simulink model "ElectricalSystem_Test"  (R2019b)
settings: Solver=VariableStepAuto  StartTime=0.0  StopTime=inf  RelTol=1e-3
PostLoadFcn:
  | set_up_test_model
undefined symbols (not defined in the file): AC1CB, AC2CB, AirSupplyIC, APSCB, ATCCabActivation, ATCZeroSpeed, ATOTBDemand, Audio, BLCB, Braking, CECB, CELCB, Class, CMCCB, CRSBCB, CSACB, CSBCB, CSCCB, DeadmanSafetyDevice, DIOCB1, DIOCB2, DLCB, DMICB, Doors, DPLCB, DRCB, EIVIB, ElectricalSystemInput, ElectricalTrainConnection, ElectricalUnitConnection, EmergencyBrakePB, Enabled, ForwardDirection, GrossMass, HasCab, HasMainCompressor, HasMotor, HasPanto, HeadlightSwitch, Height, HLCB, HornPB, ILCB1, ILCB2, IsDM1, IsDM2, IsM1, IsM2, IsT1, IsT2, LeftSideDoorOpen, Length, LoadingMass, MainReservoirPressureSwitch, MasterKeySwitch, MaxVehicles, ModeSelector, NotImmobilise, NotSafetyBrake, NVICB ... (+47)
libraries: TestBenchLib x81
(part 1 of 2)
settings Model: EnablePacing=on  Creator=jwang  LastModifiedBy=ext-nadpurob
settings DebuggingCC: FrameProcessingCompatibilityMsg=warning  ArithmeticOperatorsInVariantConditions=warning
settings SFSimCC: SimUseLocalCustomCode=off  CustomCodeUndefinedFunction=UseInterfaceOnly
settings RTWCC: RTWUseLocalCustomCode=off
settings CodeAppCC: StateflowObjectComments=on

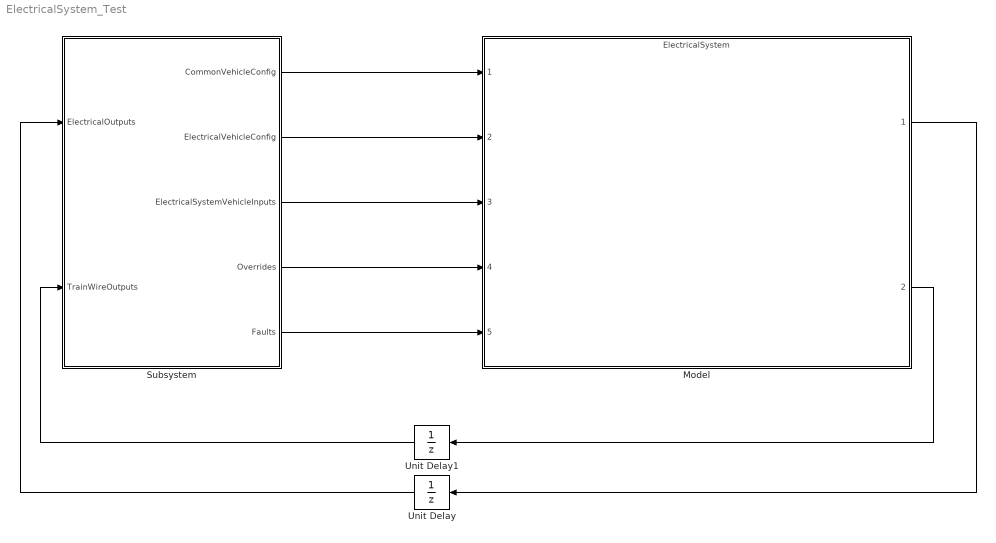
== system ElectricalSystem_Test ==
  Model : ModelReference  ModelNameDialog=ElectricalSystem.slx  ParameterArgumentNames=Prm_ElectricalSystem  ParameterArgumentValues=[Z_ElectricalSystemPrm]  UsingDefaultArgumentValue=0  SimulationMode=Normal  ModelReferenceVersion=1.1522
  Subsystem : Subsystem
  Unit Delay : UnitDelay  SampleTime=-1  HasFrameUpgradeWarning=on
  Unit Delay1 : UnitDelay  SampleTime=-1  HasFrameUpgradeWarning=on
  wires:
  Subsystem/1(CommonVehicleConfig) -> Model/1
  Subsystem/2(ElectricalVehicleConfig) -> Model/2
  Subsystem/3(ElectricalSystemVehicleInputs) -> Model/3
  Subsystem/4(Overrides) -> Model/4
  Subsystem/5(Faults) -> Model/5
  Model/2 -> Unit Delay1/1
  Model/1 -> Unit Delay/1
  Unit Delay/1 -> Subsystem/1(ElectricalOutputs)
  Unit Delay1/1 -> Subsystem/2(TrainWireOutputs)

== system ElectricalSystem_Test/Subsystem ==
  ElectricalOutputs : Inport
  TrainWireOutputs : Inport  Port=2
  Common Config Creator For Testing : Subsystem
  Data Store Memory : DataStoreMemory  DataStoreName=ElectricalSystemInput  ReadBeforeWriteMsg=warning  WriteAfterWriteMsg=warning  WriteAfterReadMsg=warning  InitialValue=zeros(1, MaxVehicles)  ShowAdditionalParam=off  OutDataTypeStr=Bus: BD_ElectricalSystem_In_Vehicle  Dimensions=MaxVehicles
  Data Store Memory1 : DataStoreMemory  DataStoreName=Faults  ReadBeforeWriteMsg=warning  WriteAfterWriteMsg=warning  WriteAfterReadMsg=warning  InitialValue=zeros(1, MaxVehicles)  ShowAdditionalParam=off  OutDataTypeStr=Bus: BD_ElectricalSystem_In_Faults  Dimensions=MaxVehicles
  Data Store Read : DataStoreRead  DataStoreName=ElectricalSystemInput
  Data Store Read1 : DataStoreRead  DataStoreName=Faults
  Data Store Write9 : DataStoreWrite  DataStoreName=ElectricalSystemInput  DataStoreElements=ElectricalSystemInput(1).ModelStatus.IsInitialized#ElectricalSystemInput(2).ModelStatus.IsInitialized#ElectricalSystemInput(3).ModelStatus.IsInitialized#ElectricalSystemInput(4).ModelStatus.IsInitialized#ElectricalSystemInput(5).ModelStatus.IsInitialized#ElectricalSystemInput(6).ModelStatus.IsInitialized
  Data Type Conversion78 : DataTypeConversion
  Electrical Config Creator For Testing : Subsystem
  Overrides1 : Subsystem
  Step : Step  SampleTime=0
  Testing : Subsystem
  CommonVehicleConfig : Outport
  ElectricalVehicleConfig : Outport  Port=2
  ElectricalSystemVehicleInputs : Outport  Port=3
  Overrides : Outport  Port=4
  Faults : Outport  Port=5
  wires:
  Common Config Creator For Testing/1(CommonVehicleConfig) -> CommonVehicleConfig/1
  Electrical Config Creator For Testing/1(ElectricalVehicleConfig) -> ElectricalVehicleConfig/1
  Overrides1/1(Override) -> Overrides/1
  Data Store Read1/1 -> Faults/1
  Data Store Read/1 -> ElectricalSystemVehicleInputs/1
  ElectricalOutputs/1 -> Testing/1(ElectricalSystemVehicleOut)
  TrainWireOutputs/1 -> Testing/2(TrainWireOutput)
  Step/1 -> Data Type Conversion78/1
  Data Type Conversion78/1 -> Data Store Write9/6, Data Store Write9/5, Data Store Write9/4, Data Store Write9/3, Data Store Write9/2, Data Store Write9/1

== system ElectricalSystem_Test/Subsystem/Common Config Creator For Testing ==
  Orientation : Constant  Value=[1 1 1 2 2 2]
  Subsystem : Subsystem
  CommonVehicleConfig : Outport  VectorParamsAs1DForOutWhenUnconnected=off
  wires:
  Orientation/1 -> Subsystem/1(Orientation)
  Subsystem/1(Out1) -> CommonVehicleConfig/1

== system ElectricalSystem_Test/Subsystem/Electrical Config Creator For Testing ==
  HasAirCompressor : Constant  Value=[1,0,0,0,0,1]  OutDataTypeStr=boolean
  HasCab : Constant  Value=[1,0,0,0,0,1]  OutDataTypeStr=boolean
  HasMotor : Constant  Value=[1,0,1,1,0,1]  OutDataTypeStr=boolean
  HasPanto : Constant  Value=[0,1,0,0,1,0]  OutDataTypeStr=boolean
  IsDM1 : Constant  Value=[1,0,0,0,0,0]  OutDataTypeStr=boolean
  IsDM2 : Constant  Value=[0,0,0,0,0,1]  OutDataTypeStr=boolean
  IsM1 : Constant  Value=[0,0,1,0,0,0]  OutDataTypeStr=boolean
  IsM2 : Constant  Value=[0,0,0,1,0,0]  OutDataTypeStr=boolean
  IsT1 : Constant  Value=[0,1,0,0,0,0]  OutDataTypeStr=boolean
  IsT2 : Constant  Value=[0,0,0,0,1,0]  OutDataTypeStr=boolean
  Subsystem : Subsystem
  ElectricalVehicleConfig : Outport  VectorParamsAs1DForOutWhenUnconnected=off
  wires:
  Subsystem/1(Out1) -> ElectricalVehicleConfig/1
  IsDM1/1 -> Subsystem/1(IsDM1)
  IsT2/1 -> Subsystem/5(isT2)
  IsDM2/1 -> Subsystem/6(IsDM2)
  HasPanto/1 -> Subsystem/7(HasPanto)
  HasCab/1 -> Subsystem/8(HasCab)
  HasMotor/1 -> Subsystem/9(HasMotor)
  HasAirCompressor/1 -> Subsystem/10(HasMainCompressor)
  IsM2/1 -> Subsystem/4(IsM2)
  IsM1/1 -> Subsystem/3(IsM1)
  IsT1/1 -> Subsystem/2(IsT1)

== system ElectricalSystem_Test/Subsystem/Overrides1 ==
  Constant : Constant  Value=zeros(1,MaxVehicles)  OutDataTypeStr=Bus: BD_ElectricalSystem_In_Overrides
  Override : Outport  VectorParamsAs1DForOutWhenUnconnected=off
  wires:
  Constant/1 -> Override/1

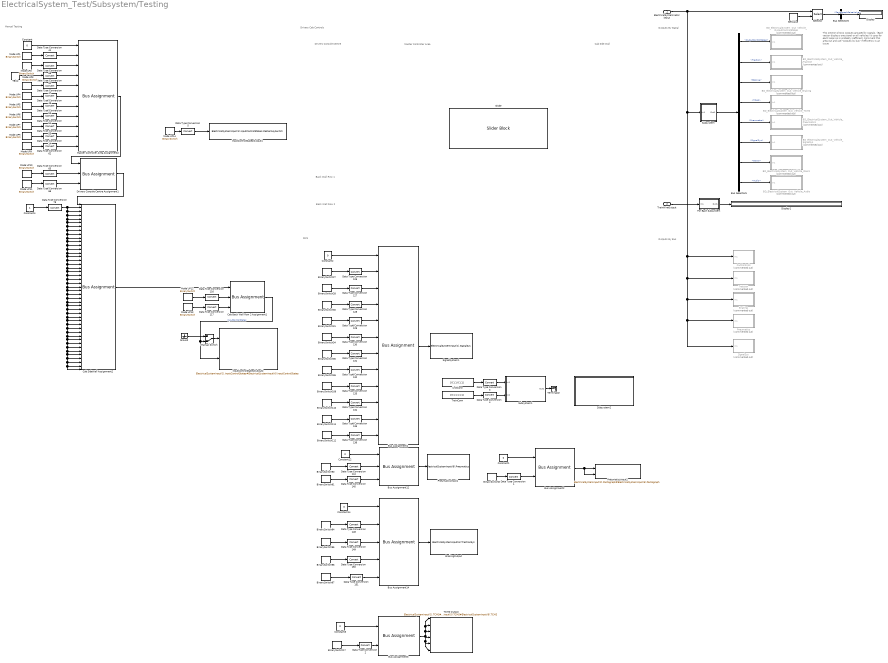
== system ElectricalSystem_Test/Subsystem/Testing ==
  note: This section shows outputs grouped by signals.
      | (Each vector displays one signal on all vehicles)
      | It uses for each loops so is probably inefficient.
      |
      | Comment this area out and use "outputs by bus" if
      | efficiency is an issue
  note: Manual Testing
  note: Outputs By Signal
  note: Drivers Cab Controls
  note: Back Wall Row 2
  note: Back Wall Row 1
  note: Cab Side Wall
  note: Drivers Console Centre
  note: Master Controller Area
  note: DM1
  note: Outputs By Bus
  ElectricalSystemVehicleOut : Inport
  TrainWireOutput : Inport  Port=2
  BD_ElectricalSystem_Out_Vehicle_Audio : Subsystem  Commented=on
  BD_ElectricalSystem_Out_Vehicle_Braking : Subsystem  Commented=on
  BD_ElectricalSystem_Out_Vehicle_Doors : Subsystem  Commented=on
  BD_ElectricalSystem_Out_Vehicle_OutputControlStates : Subsystem  Commented=on
  BD_ElectricalSystem_Out_Vehicle_Pneumatics : Subsystem  Commented=on
  BD_ElectricalSystem_Out_Vehicle_SignalSys : Subsystem  Commented=on
  BD_ElectricalSystem_Out_Vehicle_TCMS : Subsystem  Commented=on
  BD_ElectricalSystem_Out_Vehicle_Traction : Subsystem  Commented=on
  BinarySwitch{8,17,27..28,30..31,34..36,90..91,94..97,109..112} (19 alike) : TestBenchLib/BinarySwitch  value=0  init_value=0  block_colour=[0 1 0]  WorkspaceVarName=0
      settings: SourceProductName=Sydac Utilities
  Braking : Subsystem  Commented=on
  BrakingOutput : DataStoreWrite  DataStoreName=ElectricalSystemInput  DataStoreElements=ElectricalSystemInput(6).TractionSys
  Bus Assignment1 : BusAssignment  AssignedSignals=NotImmobilise,ATCZeroSpeed,NotSafetyBrake,LeftSideDoorOpen,RightSideDoorOpen,WakeUpCommand,UTOPBIndicator,UTOModeActive,ATCCabActivation,ATOTBDemand,TractionForward
  Bus Assignment12 : BusAssignment  AssignedSignals=MainReservoirPressureSwitch,PantographPressureSwitch
  Bus Assignment14 : BusAssignment  AssignedSignals=ForwardDirection,ReverseDirection,TCU_KStatus,TCU_AKStatus
  Bus Assignment2 : BusAssignment  AssignedSignals=PantographPosition
  Bus Assignment3 : BusAssignment  AssignedSignals=Overspeed
  Bus Selector5 : BusSelector  OutputSignals=OutputControlStates,Traction,Braking,TCMS,Pneumatics,SignalSys,Doors,Audio
  Bus Selector6 : BusSelector  OutputSignals=Pneumatics.PantographRaiseValve
  Cab Back Wall Row 2 Assignment1 : BusAssignment  AssignedSignals=ParkBrakeApplyPB,ParkBrakeReleasePB
  Cab SideWall Assignment2 : BusAssignment  AssignedSignals=CMCCB,RIO1CB,RIO2CB,TDICB,DIOCB2,DIOCB1,CSCCB,CSBCB,CSACB,CECB,UCCB,BLCB,CRSBCB,DMICB,NVICB,VIO1CB,VIO2CB,APSCB,DLCB,DRCB,DPLCB,HLCB,TLCB,CELCB,ILCB1,ILCB2,PANCB,TBCCB1,TBCCB2,POCB,TVDUCB,ODDCB,WFLCB,WWCB,VCBCCB,PADCB,SAC1CCB,SAC2CCB,AC1CB,AC2CB,RCCB,SFB,EIVIB,AirSupplyIC
  Constant : Constant  Value=0  OutDataTypeStr=Bus: BD_ElectricalSystem_In_Vehicle_InputControlStates
  Constant1 : Constant  Value=0  OutDataTypeStr=Bus: BD_ElectricalSystem_In_Vehicle_Pantograph
  Constant12 : Constant  Value=0  OutDataTypeStr=Bus: BD_ElectricalSystem_In_Vehicle_Pneumatics
  Constant14 : Constant  Value=0  OutDataTypeStr=Bus: BD_ElectricalSystem_In_Vehicle_Traction
  Constant2 : Constant  Value=0  OutDataTypeStr=Bus: BD_ElectricalSystem_In_Vehicle_SignalSys
  Constant3 : Constant  Value=0  OutDataTypeStr=Bus: BD_ElectricalSystem_In_Vehicle_TCMS
  Constant4 : Constant
  Data Type Conversion{1..5,14,41..42,47,49,53..55,58,62,65..66,78,116..117,126..136,144..145,148..151} (37 alike) : DataTypeConversion
  Display : Display
  Display1 : Display
  Drivers Console Centre Assignment1 : BusAssignment  AssignedSignals=EmergencyBrakePB,HornPB
  For Each Subsystem : Subsystem  TreatAsAtomicUnit=on
  Ground : Ground
  InputControlStatesOutput1 : DataStoreWrite  DataStoreName=ElectricalSystemInput  DataStoreElements=ElectricalSystemInput(1).InputControlStates.MasterKeySwitch
  InputControlStatesOutput2 : DataStoreWrite  DataStoreName=ElectricalSystemInput  DataStoreElements=ElectricalSystemInput(1).InputControlStates#ElectricalSystemInput(6).InputControlStates
  Manual Switch : ManualSwitch  CurrentSetting=0
  Master Controller Area Assignment2 : BusAssignment  AssignedSignals=MasterKeySwitch,PowerONPB,TractionBrakeController,VCBOpenPB,VCBClosePB,ParkBrakeReleasePB,DeadmanSafetyDevice,ModeSelector,WiperSwitch,HeadlightSwitch
  Mode UP{1..14} (14 alike) : TestBenchLib/BinarySwitch  value=0  init_value=0  block_colour=[0 1 0]  WorkspaceVarName=0
      settings: SourceProductName=Sydac Utilities
  OutControls : Subsystem  Commented=on
  Pneumatics : Subsystem  Commented=on
  PneumaticsInput1 : DataStoreWrite  DataStoreName=ElectricalSystemInput  DataStoreElements=ElectricalSystemInput(6).Pneumatics
  PneumaticsInput2 : DataStoreWrite  DataStoreName=ElectricalSystemInput  DataStoreElements=ElectricalSystemInput(2).Pantograph#ElectricalSystemInput(5).Pantograph
  Selector : Selector  InputPortWidth=6  IndexOptions=Index vector (port)  Indices=[1 3]  OutputSizes=1
  SetValue : TestBenchLib/SetValue  value=1  init_value=1  WorkspaceVarName=0
      settings: SourceProductName=Sydac Utilities
  SignalSys : Subsystem  Commented=on
  SignalSystem1 : DataStoreWrite  DataStoreName=ElectricalSystemInput  DataStoreElements=ElectricalSystemInput(1).SignalSys
  Slider : SliderBlock  ScaleMin=-101
  Subsystem : Subsystem
  Subsystem1 : Subsystem
  Subsystem2 : Subsystem
  TBC2 : TestBenchLib/SetValue  value=19.57995345744682  init_value=19.57995345744682  WorkspaceVarName=0
      settings: SourceProductName=Sydac Utilities
  TCMS Output : DataStoreWrite  DataStoreName=ElectricalSystemInput  DataStoreElements=ElectricalSystemInput(1).TCMS#ElectricalSystemInput(2).TCMS#ElectricalSystemInput(3).TCMS#ElectricalSystemInput(4).TCMS#ElectricalSystemInput(5).TCMS#ElectricalSystemInput(6).TCMS
  Terminator : Terminator
  Traction : Subsystem  Commented=on
  TrainConn : Constant  Value=[0 1 1 1 1 1]
  UnitConn : Constant  Value=[0 1 1 0 1 1]
  wires:
  Bus Selector5/1 -> BD_ElectricalSystem_Out_Vehicle_OutputControlStates/1(In1)  "<OutputControlStates>"
  Bus Selector5/2 -> BD_ElectricalSystem_Out_Vehicle_Traction/1(In1)  "<Traction>"
  Bus Selector5/3 -> BD_ElectricalSystem_Out_Vehicle_Braking/1(In1)  "<Braking>"
  Bus Selector5/4 -> BD_ElectricalSystem_Out_Vehicle_TCMS/1(In1)  "<TCMS>"
  Bus Selector5/5 -> BD_ElectricalSystem_Out_Vehicle_Pneumatics/1(In1)  "<Pneumatics>"
  Bus Selector5/6 -> BD_ElectricalSystem_Out_Vehicle_SignalSys/1(In1)  "<SignalSys>"
  Bus Selector5/7 -> BD_ElectricalSystem_Out_Vehicle_Doors/1(In1)  "<Doors>"
  ElectricalSystemVehicleOut/1 -> SignalSys/1(In1), Pneumatics/1(In1), Braking/1(In1), Traction/1(In1), OutControls/1(In1), Subsystem/1(In1), Selector/1
  Subsystem/1(Out1) -> Bus Selector5/1
  Master Controller Area Assignment2/1 -> Drivers Console Centre Assignment1/1
  Mode UP6/1 -> Data Type Conversion54/1
  Mode UP3/1 -> Data Type Conversion47/1
  Mode UP7/1 -> Data Type Conversion55/1
  Mode UP5/1 -> Data Type Conversion53/1
  Mode UP8/1 -> Data Type Conversion14/1
  Mode UP4/1 -> Data Type Conversion49/1
  TBC2/1 -> Data Type Conversion42/1
  Mode UP9/1 -> Data Type Conversion62/1
  Constant/1 -> Master Controller Area Assignment2/1
  Data Type Conversion41/1 -> Master Controller Area Assignment2/2
  Data Type Conversion58/1 -> Master Controller Area Assignment2/3
  Data Type Conversion42/1 -> Master Controller Area Assignment2/4
  Data Type Conversion47/1 -> Master Controller Area Assignment2/5
  Data Type Conversion49/1 -> Master Controller Area Assignment2/6
  Data Type Conversion53/1 -> Master Controller Area Assignment2/7
  Data Type Conversion54/1 -> Master Controller Area Assignment2/8
  Data Type Conversion55/1 -> Master Controller Area Assignment2/9
  Data Type Conversion14/1 -> Master Controller Area Assignment2/10
  Data Type Conversion62/1 -> Master Controller Area Assignment2/11
  Mode UP11/1 -> Data Type Conversion66/1
  Mode UP10/1 -> Data Type Conversion65/1
  Data Type Conversion65/1 -> Drivers Console Centre Assignment1/2
  Data Type Conversion66/1 -> Drivers Console Centre Assignment1/3
  Constant4/1 -> Data Type Conversion78/1
  Drivers Console Centre Assignment1/1 -> Cab SideWall Assignment2/1
  Data Type Conversion78/1 -> Cab SideWall Assignment2/3, Cab SideWall Assignment2/4, Cab SideWall Assignment2/5, Cab SideWall Assignment2/6, Cab SideWall Assignment2/7, Cab SideWall Assignment2/8, Cab SideWall Assignment2/9, Cab SideWall Assignment2/10, Cab SideWall Assignment2/11, Cab SideWall Assignment2/12, Cab SideWall Assignment2/13, Cab SideWall Assignment2/14, Cab SideWall Assignment2/15, Cab SideWall Assignment2/16, Cab SideWall Assignment2/17, Cab SideWall Assignment2/18, Cab SideWall Assignment2/19, Cab SideWall Assignment2/20, Cab SideWall Assignment2/21, Cab SideWall Assignment2/22, Cab SideWall Assignment2/23, Cab SideWall Assignment2/24, Cab SideWall Assignment2/25, Cab SideWall Assignment2/26, Cab SideWall Assignment2/27, Cab SideWall Assignment2/28, Cab SideWall Assignment2/29, Cab SideWall Assignment2/30, Cab SideWall Assignment2/31, Cab SideWall Assignment2/32, Cab SideWall Assignment2/33, Cab SideWall Assignment2/34, Cab SideWall Assignment2/35, Cab SideWall Assignment2/36, Cab SideWall Assignment2/37, Cab SideWall Assignment2/38, Cab SideWall Assignment2/39, Cab SideWall Assignment2/40, Cab SideWall Assignment2/41, Cab SideWall Assignment2/42, Cab SideWall Assignment2/43, Cab SideWall Assignment2/44, Cab SideWall Assignment2/45, Cab SideWall Assignment2/2
  Cab SideWall Assignment2/1 -> Cab Back Wall Row 2 Assignment1/1
  Mode UP13/1 -> Data Type Conversion117/1
  Mode UP12/1 -> Data Type Conversion116/1
  Cab Back Wall Row 2 Assignment1/1 -> Manual Switch/2, InputControlStatesOutput2/2  "InputControlStates"
  Data Type Conversion116/1 -> Cab Back Wall Row 2 Assignment1/2
  Data Type Conversion117/1 -> Cab Back Wall Row 2 Assignment1/3
  Constant2/1 -> Bus Assignment1/1
  BinarySwitch35/1 -> Data Type Conversion131/1
  BinarySwitch34/1 -> Data Type Conversion130/1
  BinarySwitch31/1 -> Data Type Conversion129/1
  BinarySwitch28/1 -> Data Type Conversion127/1
  BinarySwitch30/1 -> Data Type Conversion128/1
  BinarySwitch27/1 -> Data Type Conversion126/1
  Data Type Conversion126/1 -> Bus Assignment1/2
  Data Type Conversion127/1 -> Bus Assignment1/3
  Data Type Conversion128/1 -> Bus Assignment1/4
  Data Type Conversion129/1 -> Bus Assignment1/5
  Data Type Conversion130/1 -> Bus Assignment1/6
  Data Type Conversion131/1 -> Bus Assignment1/7
  BinarySwitch36/1 -> Data Type Conversion132/1
  BinarySwitch110/1 -> Data Type Conversion134/1
  BinarySwitch109/1 -> Data Type Conversion133/1
  BinarySwitch111/1 -> Data Type Conversion135/1
  BinarySwitch112/1 -> Data Type Conversion136/1
  Data Type Conversion132/1 -> Bus Assignment1/8
  Data Type Conversion133/1 -> Bus Assignment1/9
  Data Type Conversion134/1 -> Bus Assignment1/10
  Data Type Conversion135/1 -> Bus Assignment1/11
  Data Type Conversion136/1 -> Bus Assignment1/12
  Bus Assignment1/1 -> SignalSystem1/1
  Constant12/1 -> Bus Assignment12/1
  BinarySwitch90/1 -> Data Type Conversion144/1
  BinarySwitch91/1 -> Data Type Conversion145/1
  Data Type Conversion144/1 -> Bus Assignment12/2
  Data Type Conversion145/1 -> Bus Assignment12/3
  Bus Assignment12/1 -> PneumaticsInput1/1
  Constant14/1 -> Bus Assignment14/1
  BinarySwitch95/1 -> Data Type Conversion149/1
  BinarySwitch94/1 -> Data Type Conversion148/1
  Data Type Conversion148/1 -> Bus Assignment14/2
  Data Type Conversion149/1 -> Bus Assignment14/3
  BinarySwitch97/1 -> Data Type Conversion151/1
  BinarySwitch96/1 -> Data Type Conversion150/1
  Data Type Conversion150/1 -> Bus Assignment14/4
  Data Type Conversion151/1 -> Bus Assignment14/5
  Bus Assignment14/1 -> BrakingOutput/1
  SetValue/1 -> Selector/2
  Selector/1 -> Bus Selector6/1
  Bus Selector6/1 -> Display/1  "<PantographRaiseValve>"
  Bus Assignment2/1 -> PneumaticsInput2/2, PneumaticsInput2/1
  Constant1/1 -> Bus Assignment2/1
  BinarySwitch8/1 -> Data Type Conversion1/1
  Data Type Conversion1/1 -> Bus Assignment2/2
  Constant3/1 -> Bus Assignment3/1
  Bus Assignment3/1 -> TCMS Output/6, TCMS Output/5, TCMS Output/4, TCMS Output/2, TCMS Output/1, TCMS Output/3
  BinarySwitch17/1 -> Data Type Conversion2/1
  Data Type Conversion2/1 -> Bus Assignment3/2
  Bus Selector5/8 -> BD_ElectricalSystem_Out_Vehicle_Audio/1(In1)  "<Audio>"
  Manual Switch/1 -> InputControlStatesOutput2/1
  Mode UP1/1 -> Data Type Conversion41/1
  Mode UP2/1 -> Data Type Conversion58/1
  TrainWireOutput/1 -> For Each Subsystem/1(In1)
  For Each Subsystem/1(Out1) -> Display1/1
  TrainConn/1 -> Data Type Conversion4/1
  UnitConn/1 -> Data Type Conversion3/1
  Data Type Conversion3/1 -> Subsystem1/1(In1)
  Data Type Conversion4/1 -> Subsystem1/2(In2)
  Subsystem1/1(Out1) -> Terminator/1
  Data Type Conversion5/1 -> InputControlStatesOutput1/1
  Mode UP14/1 -> Data Type Conversion5/1
  Ground/1 -> Manual Switch/1

== system ElectricalSystem_Test/Subsystem/Common Config Creator For Testing/Subsystem ==
  Orientation : Inport  Partition=on  PartitionDimension=1  PartitionWidth=1  PartitionOffset=0
  Bus Assignment : BusAssignment  AssignedSignals=Enabled,Class,Orientation,Length,Height,Width,TareMass,GrossMass,LoadingMass,WheelDiameter
  Constant : Constant  Value=0  OutDataTypeStr=Bus: BD_CommonTrain_Cfg_Vehicle
  Constant1 : Constant
  Data Type Conversion : DataTypeConversion
  For Each : ForEach  DisableCoverage=on
  Ground : Ground
  Out1 : Outport  ConcatenationDimension=1  VectorParamsAs1DForOutWhenUnconnected=off
  wires:
  Constant/1 -> Bus Assignment/1
  Bus Assignment/1 -> Out1/1
  Orientation/1 -> Bus Assignment/4  "Orientation"
  Constant1/1 -> Data Type Conversion/1  "Enabled"
  Data Type Conversion/1 -> Bus Assignment/2
  Ground/1 -> Bus Assignment/11, Bus Assignment/10, Bus Assignment/9, Bus Assignment/8, Bus Assignment/7, Bus Assignment/6, Bus Assignment/5, Bus Assignment/3

== system ElectricalSystem_Test/Subsystem/Electrical Config Creator For Testing/Subsystem ==
  IsDM1 : Inport  Partition=on  PartitionDimension=1  PartitionWidth=1  PartitionOffset=0
  IsT1 : Inport  Port=2  Partition=on  PartitionDimension=1  PartitionWidth=1  PartitionOffset=0
  IsM1 : Inport  Port=3  Partition=on  PartitionDimension=1  PartitionWidth=1  PartitionOffset=0
  IsM2 : Inport  Port=4  Partition=on  PartitionDimension=1  PartitionWidth=1  PartitionOffset=0
  isT2 : Inport  Port=5  Partition=on  PartitionDimension=1  PartitionWidth=1  PartitionOffset=0
  IsDM2 : Inport  Port=6  Partition=on  PartitionDimension=1  PartitionWidth=1  PartitionOffset=0
  HasPanto : Inport  Port=7  Partition=on  PartitionDimension=1  PartitionWidth=1  PartitionOffset=0
  HasCab : Inport  Port=8  Partition=on  PartitionDimension=1  PartitionWidth=1  PartitionOffset=0
  HasMotor : Inport  Port=9  Partition=on  PartitionDimension=1  PartitionWidth=1  PartitionOffset=0
  HasMainCompressor : Inport  Port=10  Partition=on  PartitionDimension=1  PartitionWidth=1  PartitionOffset=0
  Bus Assignment : BusAssignment  AssignedSignals=IsDM1,IsT1,IsM1,IsM2,IsT2,IsDM2,HasPanto,HasCab,HasMotor,HasMainCompressor
  Constant : Constant  Value=0  OutDataTypeStr=Bus: BD_ElectricalSystem_Cfg_Vehicle
  For Each : ForEach  DisableCoverage=on
  Out1 : Outport  ConcatenationDimension=1  VectorParamsAs1DForOutWhenUnconnected=off
  wires:
  IsDM1/1 -> Bus Assignment/2
  Bus Assignment/1 -> Out1/1
  Constant/1 -> Bus Assignment/1
  IsT1/1 -> Bus Assignment/3
  IsM1/1 -> Bus Assignment/4
  IsM2/1 -> Bus Assignment/5
  isT2/1 -> Bus Assignment/6
  IsDM2/1 -> Bus Assignment/7
  HasPanto/1 -> Bus Assignment/8
  HasCab/1 -> Bus Assignment/9
  HasMotor/1 -> Bus Assignment/10
  HasMainCompressor/1 -> Bus Assignment/11

== system ElectricalSystem_Test/Subsystem/Testing/BD_ElectricalSystem_Out_Vehicle_Audio ==
  note: Tc1
  note: M1
  note: Mp1
  note: M3
  note: Mp3
  note: M2
  note: Tc2
  note: Mp2
  note: Tc1
  note: Mp1
  note: M1
  note: Mp3
  note: M3
  note: M2
  note: Mp2
  note: Tc2
  In1 : Inport
  ExtractData : Subsystem  TreatAsAtomicUnit=on
  Pwr{,1..3} (4 alike) : Display
  wires:
  In1/1 -> ExtractData/1(In1)
  ExtractData/1(Out1) -> Pwr/1
  ExtractData/2(Out2) -> Pwr1/1
  ExtractData/3(Out3) -> Pwr2/1
  ExtractData/4(Out4) -> Pwr3/1

== system ElectricalSystem_Test/Subsystem/Testing/BD_ElectricalSystem_Out_Vehicle_Braking ==
  note: ScopyBois
  note: Tc1
  note: Mp1
  note: M1
  note: Mp3
  note: M3
  note: M2
  note: Mp2
  note: Tc2
  note: Tc1
  note: Mp1
  note: M1
  note: Mp3
  note: M3
  note: M2
  note: Mp2
  note: Tc2
  In1 : Inport
  ExtractData : Subsystem  TreatAsAtomicUnit=on
  Pwr{,1..3,6..9} (8 alike) : Display
  wires:
  ExtractData/1(Power) -> Pwr/1
  In1/1 -> ExtractData/1(In1)
  ExtractData/2(Traction) -> Pwr1/1
  ExtractData/3(Braking) -> Pwr2/1
  ExtractData/4(Not High Braking) -> Pwr3/1
  ExtractData/5(Force Brake Release Cmd) -> Pwr6/1
  ExtractData/6(Backup Mode) -> Pwr7/1
  ExtractData/7(NoEB) -> Pwr8/1
  ExtractData/8(NoEB1) -> Pwr9/1

== system ElectricalSystem_Test/Subsystem/Testing/BD_ElectricalSystem_Out_Vehicle_Doors ==
  note: Tc2
  note: Mp2
  note: M2
  note: M3
  note: Mp3
  note: M1
  note: Mp1
  note: Tc1
  note: Mp2
  note: Tc2
  note: M2
  note: Mp3
  note: M3
  note: Mp1
  note: M1
  note: Tc1
  In1 : Inport
  ExtractData : Subsystem  TreatAsAtomicUnit=on
  Pwr{,1..7} (8 alike) : Display
  wires:
  ExtractData/8(Out8) -> Pwr7/1
  ExtractData/7(Out7) -> Pwr6/1
  ExtractData/6(Out6) -> Pwr5/1
  ExtractData/5(Out5) -> Pwr4/1
  ExtractData/4(Out4) -> Pwr3/1
  ExtractData/3(Out3) -> Pwr2/1
  ExtractData/2(Out2) -> Pwr1/1
  ExtractData/1(Out1) -> Pwr/1
  In1/1 -> ExtractData/1(In1)

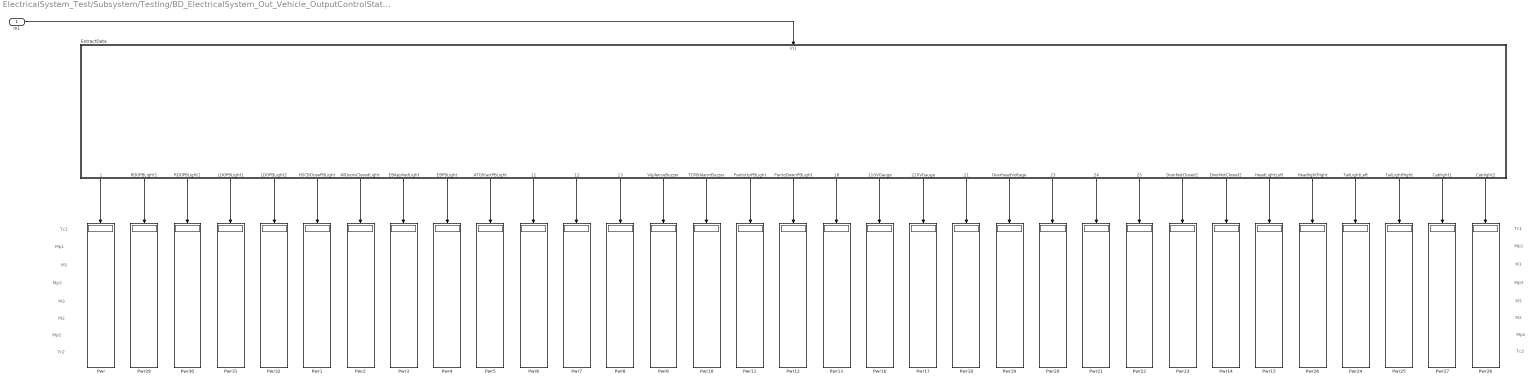
== system ElectricalSystem_Test/Subsystem/Testing/BD_ElectricalSystem_Out_Vehicle_OutputControlStates ==
  note: Tc1
  note: M1
  note: Mp1
  note: M3
  note: Mp3
  note: M2
  note: Tc2
  note: Mp2
  note: Tc1
  note: Mp1
  note: M1
  note: Mp3
  note: M3
  note: M2
  note: Mp2
  note: Tc2
  In1 : Inport
  ExtractData : Subsystem  TreatAsAtomicUnit=on
  Pwr{,1..32} (33 alike) : Display
  wires:
  ExtractData/16(PantoUpPBLight) -> Pwr11/1
  ExtractData/15(TCMSAlarmBuzzer) -> Pwr10/1
  ExtractData/14(VigilanceBuzzer) -> Pwr9/1
  ExtractData/13(DualPressureGaugeBacklight) -> Pwr8/1
  ExtractData/12(BrakeCylinderPressureGauge) -> Pwr7/1
  ExtractData/11(MainReservoirPipePressureGauge) -> Pwr6/1
  ExtractData/10(ATOStartPBLight) -> Pwr5/1
  ExtractData/9(EBPBLight) -> Pwr4/1
  ExtractData/8(EBAppliedLight) -> Pwr3/1
  ExtractData/7(AllDoorsClosedLight) -> Pwr2/1
  ExtractData/6(HSCBClosePBLight) -> Pwr1/1
  ExtractData/1(AutomaticChangeEndPBLight) -> Pwr/1
  In1/1 -> ExtractData/1(In1)
  ExtractData/18(ParkBrakeApplyPBLight) -> Pwr13/1
  ExtractData/19(110VGauge) -> Pwr16/1
  ExtractData/20(220VGauge) -> Pwr17/1
  ExtractData/21(DualBatteryGaugeBacklight) -> Pwr18/1
  ExtractData/22(OverheadVoltage) -> Pwr19/1
  ExtractData/23(OverheadVoltageBacklight) -> Pwr20/1
  ExtractData/24(PneumaticBrakesNotReleased1) -> Pwr21/1
  ExtractData/25(PneumaticBrakesNotReleased2) -> Pwr22/1
  ExtractData/26(DoorNotClosed1) -> Pwr23/1
  ExtractData/27(DoorNotClosed2) -> Pwr14/1
  ExtractData/28(HeadLightLeft) -> Pwr15/1
  ExtractData/29(HeadlightRight) -> Pwr26/1
  ExtractData/30(TailLightLeft) -> Pwr24/1
  ExtractData/17(PantoDownPBLight) -> Pwr12/1
  ExtractData/31(TailLightRight) -> Pwr25/1
  ExtractData/32(Cablight1) -> Pwr27/1
  ExtractData/33(Cablight2) -> Pwr28/1
  ExtractData/2(RDOPBLight1) -> Pwr29/1
  ExtractData/3(RDOPBLight2) -> Pwr30/1
  ExtractData/4(LDOPBLight1) -> Pwr31/1
  ExtractData/5(LDOPBLight2) -> Pwr32/1

== system ElectricalSystem_Test/Subsystem/Testing/BD_ElectricalSystem_Out_Vehicle_Pneumatics ==
  note: Tc2
  note: Mp2
  note: M2
  note: M3
  note: Mp3
  note: M1
  note: Mp1
  note: Tc1
  note: Mp2
  note: Tc2
  note: M2
  note: Mp3
  note: M3
  note: Mp1
  note: M1
  note: Tc1
  In1 : Inport
  ExtractData : Subsystem  TreatAsAtomicUnit=on
  Pwr{,1..4} (5 alike) : Display
  wires:
  ExtractData/5(Out3) -> Pwr2/1
  ExtractData/2(Out2) -> Pwr1/1
  ExtractData/1(Out1) -> Pwr/1
  In1/1 -> ExtractData/1(In1)
  ExtractData/3(Out4) -> Pwr3/1
  ExtractData/4(Out5) -> Pwr4/1

== system ElectricalSystem_Test/Subsystem/Testing/BD_ElectricalSystem_Out_Vehicle_SignalSys ==
  note: Tc1
  note: M1
  note: Mp1
  note: M3
  note: Mp3
  note: M2
  note: Tc2
  note: Mp2
  note: Tc1
  note: Mp1
  note: M1
  note: Mp3
  note: M3
  note: M2
  note: Mp2
  note: Tc2
  In1 : Inport
  ExtractData : Subsystem  TreatAsAtomicUnit=on
  Pwr{,1..18} (19 alike) : Display
  wires:
  In1/1 -> ExtractData/1(In1)
  ExtractData/1(Out1) -> Pwr/1
  ExtractData/2(Out2) -> Pwr1/1
  ExtractData/3(Out3) -> Pwr2/1
  ExtractData/4(Out4) -> Pwr3/1
  ExtractData/5(Out5) -> Pwr4/1
  ExtractData/6(Out6) -> Pwr5/1
  ExtractData/7(Out7) -> Pwr6/1
  ExtractData/8(Out8) -> Pwr7/1
  ExtractData/9(Out9) -> Pwr8/1
  ExtractData/10(Out10) -> Pwr9/1
  ExtractData/11(Out11) -> Pwr10/1
  ExtractData/12(Out12) -> Pwr11/1
  ExtractData/13(Out13) -> Pwr12/1
  ExtractData/14(Out14) -> Pwr13/1
  ExtractData/15(Out15) -> Pwr14/1
  ExtractData/16(Out16) -> Pwr15/1
  ExtractData/17(Out17) -> Pwr16/1
  ExtractData/18(Out18) -> Pwr17/1
  ExtractData/19(Out19) -> Pwr18/1

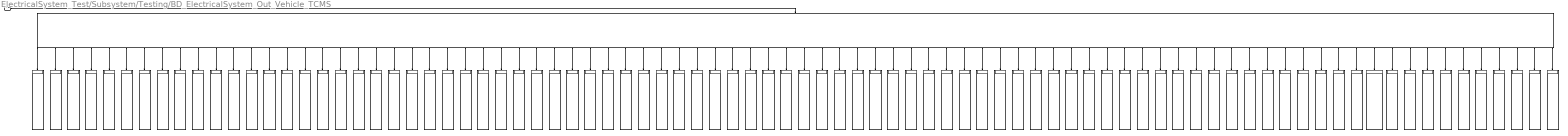
== system ElectricalSystem_Test/Subsystem/Testing/BD_ElectricalSystem_Out_Vehicle_TCMS ==
  note: Tc1
  note: M1
  note: Mp1
  note: M3
  note: Mp3
  note: M2
  note: Tc2
  note: Mp2
  note: Tc1
  note: Mp1
  note: M1
  note: Mp3
  note: M3
  note: M2
  note: Mp2
  note: Tc2
  In1 : Inport
  ExtractData : Subsystem  TreatAsAtomicUnit=on
  Pwr{,1..85} (86 alike) : Display
  wires:
  In1/1 -> ExtractData/1(In1)
  ExtractData/2(Out1) -> Pwr63/1
  ExtractData/3(Out2) -> Pwr1/1
  ExtractData/4(Out3) -> Pwr2/1
  ExtractData/5(Out4) -> Pwr3/1
  ExtractData/6(Out5) -> Pwr4/1
  ExtractData/7(Out6) -> Pwr5/1
  ExtractData/8(Out7) -> Pwr6/1
  ExtractData/9(Out8) -> Pwr7/1
  ExtractData/10(Out9) -> Pwr8/1
  ExtractData/11(Out10) -> Pwr9/1
  ExtractData/12(Out11) -> Pwr10/1
  ExtractData/13(Out12) -> Pwr11/1
  ExtractData/14(Out13) -> Pwr12/1
  ExtractData/15(Out14) -> Pwr13/1
  ExtractData/16(Out15) -> Pwr14/1
  ExtractData/17(Out16) -> Pwr15/1
  ExtractData/18(Out17) -> Pwr16/1
  ExtractData/19(Out18) -> Pwr17/1
  ExtractData/20(Out19) -> Pwr18/1
  ExtractData/21(Out20) -> Pwr19/1
  ExtractData/22(Out21) -> Pwr20/1
  ExtractData/23(Out22) -> Pwr21/1
  ExtractData/24(Out23) -> Pwr22/1
  ExtractData/25(Out24) -> Pwr23/1
  ExtractData/26(Out25) -> Pwr24/1
  ExtractData/27(Out26) -> Pwr25/1
  ExtractData/28(Out27) -> Pwr26/1
  ExtractData/29(Out28) -> Pwr27/1
  ExtractData/30(Out29) -> Pwr28/1
  ExtractData/31(Out30) -> Pwr29/1
  ExtractData/32(Out31) -> Pwr30/1
  ExtractData/33(Out32) -> Pwr41/1
  ExtractData/34(Out33) -> Pwr51/1
  ExtractData/35(Out34) -> Pwr52/1
  ExtractData/36(Out35) -> Pwr53/1
  ExtractData/37(Out36) -> Pwr54/1
  ExtractData/38(Out37) -> Pwr55/1
  ExtractData/39(Out38) -> Pwr56/1
  ExtractData/40(Out39) -> Pwr57/1
  ExtractData/41(Out40) -> Pwr31/1
  ExtractData/42(Out41) -> Pwr32/1
  ExtractData/43(Out42) -> Pwr33/1
  ExtractData/44(Out43) -> Pwr34/1
  ExtractData/45(Out44) -> Pwr35/1
  ExtractData/46(Out45) -> Pwr36/1
  ExtractData/47(Out46) -> Pwr37/1
  ExtractData/48(Out47) -> Pwr38/1
  ExtractData/49(Out48) -> Pwr39/1
  ExtractData/50(Out49) -> Pwr40/1
  ExtractData/51(Out50) -> Pwr42/1
  ExtractData/52(Out51) -> Pwr43/1
  ExtractData/53(Out52) -> Pwr44/1
  ExtractData/54(Out53) -> Pwr45/1
  ExtractData/55(Out54) -> Pwr46/1
  ExtractData/56(Out55) -> Pwr47/1
  ExtractData/57(Out56) -> Pwr48/1
  ExtractData/58(Out57) -> Pwr49/1
  ExtractData/59(Out58) -> Pwr50/1
  ExtractData/60(Out59) -> Pwr58/1
  ExtractData/61(Out60) -> Pwr59/1
  ExtractData/62(Out61) -> Pwr60/1
  ExtractData/63(Out62) -> Pwr61/1
  ExtractData/64(Out63) -> Pwr62/1
  ExtractData/65(Out65) -> Pwr64/1
  ExtractData/66(Out66) -> Pwr65/1
  ExtractData/67(Out67) -> Pwr66/1
  ExtractData/68(Out68) -> Pwr67/1
  ExtractData/69(Out69) -> Pwr68/1
  ExtractData/70(Out70) -> Pwr69/1
  ExtractData/71(Out71) -> Pwr70/1
  ExtractData/72(Out72) -> Pwr71/1
  ExtractData/73(Out73) -> Pwr72/1
  ExtractData/74(Out74) -> Pwr73/1
  ExtractData/75(Out75) -> Pwr74/1
  ExtractData/76(Out76) -> Pwr75/1
  ExtractData/77(Out77) -> Pwr76/1
  ExtractData/78(Out78) -> Pwr77/1
  ExtractData/79(Out79) -> Pwr78/1
  ExtractData/80(Out80) -> Pwr79/1
  ExtractData/81(Out81) -> Pwr80/1
  ExtractData/82(Out82) -> Pwr81/1
  ExtractData/83(Out83) -> Pwr82/1
  ExtractData/84(Out84) -> Pwr83/1
  ExtractData/85(Out85) -> Pwr84/1
  ExtractData/1(Out64) -> Pwr/1
  ExtractData/86(Out86) -> Pwr85/1

== system ElectricalSystem_Test/Subsystem/Testing/BD_ElectricalSystem_Out_Vehicle_Traction ==
  note: Tc2
  note: Mp2
  note: M2
  note: M3
  note: Mp3
  note: M1
  note: Mp1
  note: Tc1
  note: Mp2
  note: Tc2
  note: M2
  note: Mp3
  note: M3
  note: Mp1
  note: M1
  note: Tc1
  In1 : Inport
  ExtractData : Subsystem  TreatAsAtomicUnit=on
  Pwr{,1..15} (16 alike) : Display
  wires:
  In1/1 -> ExtractData/1(In1)
  ExtractData/1(Out) -> Pwr/1
  ExtractData/2(Out1) -> Pwr1/1
  ExtractData/3(Out2) -> Pwr2/1
  ExtractData/4(Out3) -> Pwr3/1
  ExtractData/5(Out4) -> Pwr4/1
  ExtractData/6(Out5) -> Pwr5/1
  ExtractData/7(Out6) -> Pwr6/1
  ExtractData/8(Out7) -> Pwr7/1
  ExtractData/9(Out8) -> Pwr8/1
  ExtractData/10(Out9) -> Pwr9/1
  ExtractData/11(Out10) -> Pwr10/1
  ExtractData/12(Out11) -> Pwr11/1
  ExtractData/13(Out12) -> Pwr12/1
  ExtractData/14(Out13) -> Pwr13/1
  ExtractData/16(Out15) -> Pwr15/1
  ExtractData/15(Out14) -> Pwr14/1

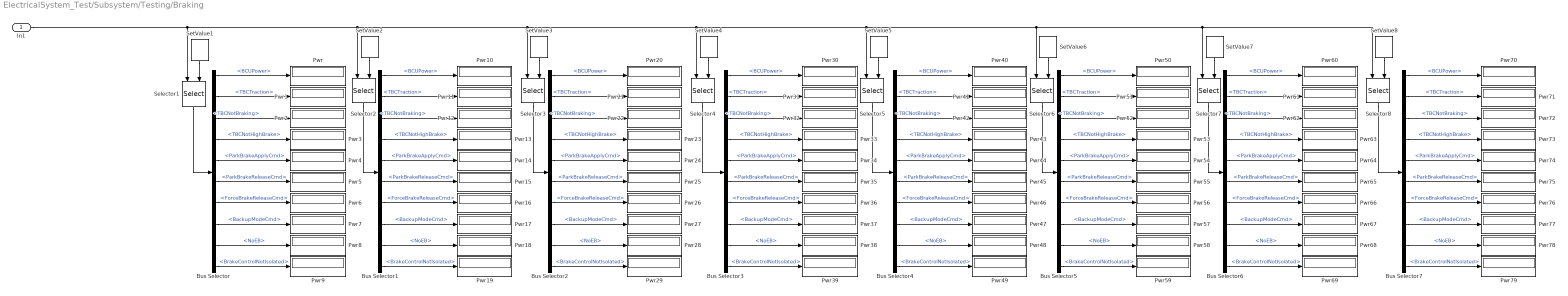
== system ElectricalSystem_Test/Subsystem/Testing/Braking ==
  In1 : Inport
  Bus Selector{,1..7} (8 alike) : BusSelector  OutputSignals=Braking.BCUPower,Braking.TBCTraction,Braking.TBCNotBraking,Braking.TBCNotHighBrake,Pneumatics.ParkBrakeApplyCmd,Pneumatics.ParkBrakeReleaseCmd,Braking.ForceBrakeReleaseCmd,Braking.BackupModeCmd,Braking.NoEB,Braking.BrakeControlNotIsolated
  Pwr{,1..79} (80 alike) : Display
  Selector{1..8} (8 alike) : Selector  InputPortWidth=8  IndexOptions=Index vector (port)  Indices=[1 3]  OutputSizes=1
  SetValue1 : TestBenchLib/SetValue  value=1  init_value=1  WorkspaceVarName=0
      settings: SourceProductName=Sydac Utilities
  SetValue2 : TestBenchLib/SetValue  value=2  init_value=2  WorkspaceVarName=0
      settings: SourceProductName=Sydac Utilities
  SetValue3 : TestBenchLib/SetValue  value=3  init_value=3  WorkspaceVarName=0
      settings: SourceProductName=Sydac Utilities
  SetValue4 : TestBenchLib/SetValue  value=4  init_value=4  WorkspaceVarName=0
      settings: SourceProductName=Sydac Utilities
  SetValue5 : TestBenchLib/SetValue  value=5  init_value=5  WorkspaceVarName=0
      settings: SourceProductName=Sydac Utilities
  SetValue6 : TestBenchLib/SetValue  value=6  init_value=6  WorkspaceVarName=0
      settings: SourceProductName=Sydac Utilities
  SetValue7 : TestBenchLib/SetValue  value=7  init_value=7  WorkspaceVarName=0
      settings: SourceProductName=Sydac Utilities
  SetValue8 : TestBenchLib/SetValue  value=8  init_value=8  WorkspaceVarName=0
      settings: SourceProductName=Sydac Utilities
  wires:
  Selector1/1 -> Bus Selector/1
  SetValue1/1 -> Selector1/2
  Bus Selector/1 -> Pwr/1  "<BCUPower>"
  Bus Selector/2 -> Pwr1/1  "<TBCTraction>"
  Bus Selector/3 -> Pwr2/1  "<TBCNotBraking>"
  Bus Selector/4 -> Pwr3/1  "<TBCNotHighBrake>"
  Bus Selector/5 -> Pwr4/1  "<ParkBrakeApplyCmd>"
  Bus Selector/6 -> Pwr5/1  "<ParkBrakeReleaseCmd>"
  Bus Selector/7 -> Pwr6/1  "<ForceBrakeReleaseCmd>"
  Bus Selector/8 -> Pwr7/1  "<BackupModeCmd>"
  Bus Selector/9 -> Pwr8/1  "<NoEB>"
  Bus Selector/10 -> Pwr9/1  "<BrakeControlNotIsolated>"
  Selector2/1 -> Bus Selector1/1
  SetValue2/1 -> Selector2/2
  SetValue3/1 -> Selector3/2
  SetValue4/1 -> Selector4/2
  SetValue5/1 -> Selector5/2
  In1/1 -> Selector8/1, Selector7/1, Selector6/1, Selector5/1, Selector4/1, Selector3/1, Selector2/1, Selector1/1
  SetValue6/1 -> Selector6/2
  SetValue7/1 -> Selector7/2
  SetValue8/1 -> Selector8/2
  Bus Selector1/10 -> Pwr19/1  "<BrakeControlNotIsolated>"
  Bus Selector1/9 -> Pwr18/1  "<NoEB>"
  Bus Selector1/8 -> Pwr17/1  "<BackupModeCmd>"
  Bus Selector1/7 -> Pwr16/1  "<ForceBrakeReleaseCmd>"
  Bus Selector1/6 -> Pwr15/1  "<ParkBrakeReleaseCmd>"
  Bus Selector1/5 -> Pwr14/1  "<ParkBrakeApplyCmd>"
  Bus Selector1/4 -> Pwr13/1  "<TBCNotHighBrake>"
  Bus Selector1/3 -> Pwr12/1  "<TBCNotBraking>"
  Bus Selector1/2 -> Pwr11/1  "<TBCTraction>"
  Bus Selector1/1 -> Pwr10/1  "<BCUPower>"
  Bus Selector2/1 -> Pwr20/1  "<BCUPower>"
  Bus Selector2/2 -> Pwr21/1  "<TBCTraction>"
  Bus Selector2/3 -> Pwr22/1  "<TBCNotBraking>"
  Bus Selector2/4 -> Pwr23/1  "<TBCNotHighBrake>"
  Bus Selector2/5 -> Pwr24/1  "<ParkBrakeApplyCmd>"
  Bus Selector2/6 -> Pwr25/1  "<ParkBrakeReleaseCmd>"
  Bus Selector2/7 -> Pwr26/1  "<ForceBrakeReleaseCmd>"
  Bus Selector2/8 -> Pwr27/1  "<BackupModeCmd>"
  Bus Selector2/9 -> Pwr28/1  "<NoEB>"
  Bus Selector2/10 -> Pwr29/1  "<BrakeControlNotIsolated>"
  Bus Selector3/10 -> Pwr39/1  "<BrakeControlNotIsolated>"
  Bus Selector3/9 -> Pwr38/1  "<NoEB>"
  Bus Selector3/8 -> Pwr37/1  "<BackupModeCmd>"
  Bus Selector3/7 -> Pwr36/1  "<ForceBrakeReleaseCmd>"
  Bus Selector3/6 -> Pwr35/1  "<ParkBrakeReleaseCmd>"
  Bus Selector3/5 -> Pwr34/1  "<ParkBrakeApplyCmd>"
  Bus Selector3/4 -> Pwr33/1  "<TBCNotHighBrake>"
  Bus Selector3/3 -> Pwr32/1  "<TBCNotBraking>"
  Bus Selector3/2 -> Pwr31/1  "<TBCTraction>"
  Bus Selector3/1 -> Pwr30/1  "<BCUPower>"
  Bus Selector4/1 -> Pwr40/1  "<BCUPower>"
  Bus Selector4/2 -> Pwr41/1  "<TBCTraction>"
  Bus Selector4/3 -> Pwr42/1  "<TBCNotBraking>"
  Bus Selector4/4 -> Pwr43/1  "<TBCNotHighBrake>"
  Bus Selector4/5 -> Pwr44/1  "<ParkBrakeApplyCmd>"
  Bus Selector4/6 -> Pwr45/1  "<ParkBrakeReleaseCmd>"
  Bus Selector4/7 -> Pwr46/1  "<ForceBrakeReleaseCmd>"
  Bus Selector4/8 -> Pwr47/1  "<BackupModeCmd>"
  Bus Selector4/9 -> Pwr48/1  "<NoEB>"
  Bus Selector4/10 -> Pwr49/1  "<BrakeControlNotIsolated>"
  Bus Selector5/10 -> Pwr59/1  "<BrakeControlNotIsolated>"
  Bus Selector5/9 -> Pwr58/1  "<NoEB>"
  Bus Selector5/8 -> Pwr57/1  "<BackupModeCmd>"
  Bus Selector5/7 -> Pwr56/1  "<ForceBrakeReleaseCmd>"
  Bus Selector5/6 -> Pwr55/1  "<ParkBrakeReleaseCmd>"
  Bus Selector5/5 -> Pwr54/1  "<ParkBrakeApplyCmd>"
  Bus Selector5/4 -> Pwr53/1  "<TBCNotHighBrake>"
  Bus Selector5/3 -> Pwr52/1  "<TBCNotBraking>"
  Bus Selector5/2 -> Pwr51/1  "<TBCTraction>"
  Bus Selector5/1 -> Pwr50/1  "<BCUPower>"
  Bus Selector6/1 -> Pwr60/1  "<BCUPower>"
  Bus Selector6/2 -> Pwr61/1  "<TBCTraction>"
  Bus Selector6/3 -> Pwr62/1  "<TBCNotBraking>"
  Bus Selector6/4 -> Pwr63/1  "<TBCNotHighBrake>"
  Bus Selector6/5 -> Pwr64/1  "<ParkBrakeApplyCmd>"
  Bus Selector6/6 -> Pwr65/1  "<ParkBrakeReleaseCmd>"
  Bus Selector6/7 -> Pwr66/1  "<ForceBrakeReleaseCmd>"
  Bus Selector6/8 -> Pwr67/1  "<BackupModeCmd>"
  Bus Selector6/9 -> Pwr68/1  "<NoEB>"
  Bus Selector6/10 -> Pwr69/1  "<BrakeControlNotIsolated>"
  Bus Selector7/10 -> Pwr79/1  "<BrakeControlNotIsolated>"
  Bus Selector7/9 -> Pwr78/1  "<NoEB>"
  Bus Selector7/8 -> Pwr77/1  "<BackupModeCmd>"
  Bus Selector7/7 -> Pwr76/1  "<ForceBrakeReleaseCmd>"
  Bus Selector7/6 -> Pwr75/1  "<ParkBrakeReleaseCmd>"
  Bus Selector7/5 -> Pwr74/1  "<ParkBrakeApplyCmd>"
  Bus Selector7/4 -> Pwr73/1  "<TBCNotHighBrake>"
  Bus Selector7/3 -> Pwr72/1  "<TBCNotBraking>"
  Bus Selector7/2 -> Pwr71/1  "<TBCTraction>"
  Bus Selector7/1 -> Pwr70/1  "<BCUPower>"
  Selector3/1 -> Bus Selector2/1
  Selector4/1 -> Bus Selector3/1
  Selector6/1 -> Bus Selector5/1
  Selector7/1 -> Bus Selector6/1
  Selector8/1 -> Bus Selector7/1
  Selector5/1 -> Bus Selector4/1

== system ElectricalSystem_Test/Subsystem/Testing/For Each Subsystem ==
  In1 : Inport  Partition=on  PartitionDimension=1  PartitionWidth=1  PartitionOffset=0
  Bus Selector : BusSelector  OutputSignals=TrainWires.TW31102
  For Each : ForEach  DisableCoverage=on
  Out1 : Outport  ConcatenationDimension=1
  wires:
  In1/1 -> Bus Selector/1
  Bus Selector/1 -> Out1/1  "<TW31102>"

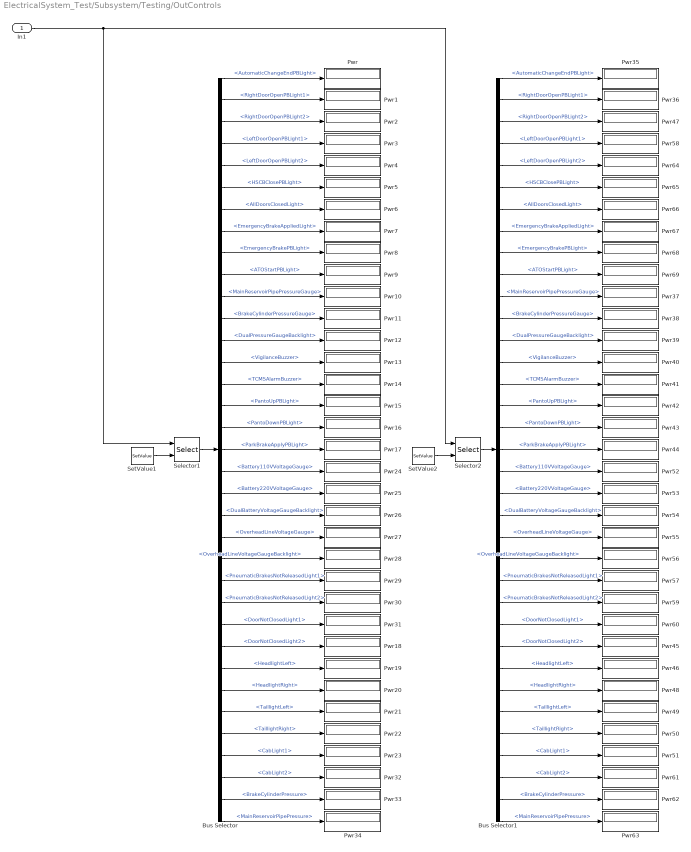
== system ElectricalSystem_Test/Subsystem/Testing/OutControls ==
  In1 : Inport
  Bus Selector : BusSelector  OutputSignals=OutputControlStates.AutomaticChangeEndPBLight,OutputControlStates.RightDoorOpenPBLight1,OutputControlStates.RightDoorOpenPBLight2,OutputControlStates.LeftDoorOpenPBLight1,OutputControlStates.LeftDoorOpenPBLight2,OutputControlStates.HSCBClosePBLight,OutputControlStates.AllDoorsClosedLight,OutputControlStates.EmergencyBrakeAppliedLight,OutputControlStates.EmergencyBrakePBLight,OutputControlStates.ATOStartPBLight,OutputControlStates.MainReservoirPipePressureGauge,OutputControlStates.BrakeCylinderPressureGauge,OutputControlStates.DualPressureGaugeBacklight,OutputControlStates.VigilanceBuzzer,OutputControlStates.TCMSAlarmBuzzer,OutputControlStates.PantoUpPBLight,OutputControlStates.PantoDownPBLight,OutputControlStates.ParkBrakeApplyPBLight,OutputControlStates.Battery110VVoltageGauge,OutputControlStates.Battery220VVoltageGauge,OutputControlStates.DualBatteryVoltageGaugeBacklight,OutputControlStates.OverheadLineVoltageGauge,OutputControlStates.OverheadLineVoltageGaugeBacklight,OutputControlStates.PneumaticBrakesNotReleasedLight1,OutputControlStates.PneumaticBrakesNotReleasedLight2,OutputControlStates.DoorNotClosedLight1,OutputControlStates.DoorNotClosedLight2,OutputControlStates.HeadlightLeft,OutputControlStates.HeadlightRight,OutputControlStates.TaillightLeft,OutputControlStates.TaillightRight,OutputControlStates.CabLight1,OutputControlStates.CabLight2,OutputControlStates.BrakeCylinderPressure,OutputControlStates.MainReservoirPipePressure
  Bus Selector1 : BusSelector  OutputSignals=OutputControlStates.AutomaticChangeEndPBLight,OutputControlStates.RightDoorOpenPBLight1,OutputControlStates.RightDoorOpenPBLight2,OutputControlStates.LeftDoorOpenPBLight1,OutputControlStates.LeftDoorOpenPBLight2,OutputControlStates.HSCBClosePBLight,OutputControlStates.AllDoorsClosedLight,OutputControlStates.EmergencyBrakeAppliedLight,OutputControlStates.EmergencyBrakePBLight,OutputControlStates.ATOStartPBLight,OutputControlStates.MainReservoirPipePressureGauge,OutputControlStates.BrakeCylinderPressureGauge,OutputControlStates.DualPressureGaugeBacklight,OutputControlStates.VigilanceBuzzer,OutputControlStates.TCMSAlarmBuzzer,OutputControlStates.PantoUpPBLight,OutputControlStates.PantoDownPBLight,OutputControlStates.ParkBrakeApplyPBLight,OutputControlStates.Battery110VVoltageGauge,OutputControlStates.Battery220VVoltageGauge,OutputControlStates.DualBatteryVoltageGaugeBacklight,OutputControlStates.OverheadLineVoltageGauge,OutputControlStates.OverheadLineVoltageGaugeBacklight,OutputControlStates.PneumaticBrakesNotReleasedLight1,OutputControlStates.PneumaticBrakesNotReleasedLight2,OutputControlStates.DoorNotClosedLight1,OutputControlStates.DoorNotClosedLight2,OutputControlStates.HeadlightLeft,OutputControlStates.HeadlightRight,OutputControlStates.TaillightLeft,OutputControlStates.TaillightRight,OutputControlStates.CabLight1,OutputControlStates.CabLight2,OutputControlStates.BrakeCylinderPressure,OutputControlStates.MainReservoirPipePressure
  Pwr{,1..69} (70 alike) : Display
  Selector1 : Selector  InputPortWidth=8  IndexOptions=Index vector (port)  Indices=[1 3]  OutputSizes=1
  Selector2 : Selector  InputPortWidth=8  IndexOptions=Index vector (port)  Indices=[1 3]  OutputSizes=1
  SetValue1 : TestBenchLib/SetValue  value=1  init_value=1  WorkspaceVarName=0
      settings: SourceProductName=Sydac Utilities
  SetValue2 : TestBenchLib/SetValue  value=8  init_value=8  WorkspaceVarName=0
      settings: SourceProductName=Sydac Utilities
  wires:
  In1/1 -> Selector2/1, Selector1/1
  SetValue1/1 -> Selector1/2
  Selector1/1 -> Bus Selector/1
  Bus Selector/1 -> Pwr/1  "<AutomaticChangeEndPBLight>"
  Bus Selector/2 -> Pwr1/1  "<RightDoorOpenPBLight1>"
  Bus Selector/3 -> Pwr2/1  "<RightDoorOpenPBLight2>"
  Bus Selector/4 -> Pwr3/1  "<LeftDoorOpenPBLight1>"
  Bus Selector/5 -> Pwr4/1  "<LeftDoorOpenPBLight2>"
  Bus Selector/6 -> Pwr5/1  "<HSCBClosePBLight>"
  Bus Selector/7 -> Pwr6/1  "<AllDoorsClosedLight>"
  Bus Selector/8 -> Pwr7/1  "<EmergencyBrakeAppliedLight>"
  Bus Selector/9 -> Pwr8/1  "<EmergencyBrakePBLight>"
  Bus Selector/10 -> Pwr9/1  "<ATOStartPBLight>"
  Bus Selector/11 -> Pwr10/1  "<MainReservoirPipePressureGauge>"
  Bus Selector/12 -> Pwr11/1  "<BrakeCylinderPressureGauge>"
  Bus Selector/13 -> Pwr12/1  "<DualPressureGaugeBacklight>"
  Bus Selector/14 -> Pwr13/1  "<VigilanceBuzzer>"
  Bus Selector/15 -> Pwr14/1  "<TCMSAlarmBuzzer>"
  Bus Selector/16 -> Pwr15/1  "<PantoUpPBLight>"
  Bus Selector/17 -> Pwr16/1  "<PantoDownPBLight>"
  Bus Selector/18 -> Pwr17/1  "<ParkBrakeApplyPBLight>"
  Bus Selector/19 -> Pwr24/1  "<Battery110VVoltageGauge>"
  Bus Selector/20 -> Pwr25/1  "<Battery220VVoltageGauge>"
  Bus Selector/21 -> Pwr26/1  "<DualBatteryVoltageGaugeBacklight>"
  Bus Selector/22 -> Pwr27/1  "<OverheadLineVoltageGauge>"
  Bus Selector/23 -> Pwr28/1  "<OverheadLineVoltageGaugeBacklight>"
  Bus Selector/24 -> Pwr29/1  "<PneumaticBrakesNotReleasedLight1>"
  Bus Selector/25 -> Pwr30/1  "<PneumaticBrakesNotReleasedLight2>"
  Bus Selector/26 -> Pwr31/1  "<DoorNotClosedLight1>"
  Bus Selector/27 -> Pwr18/1  "<DoorNotClosedLight2>"
  Bus Selector/28 -> Pwr19/1  "<HeadlightLeft>"
  Bus Selector/29 -> Pwr20/1  "<HeadlightRight>"
  Bus Selector/30 -> Pwr21/1  "<TaillightLeft>"
  Bus Selector/31 -> Pwr22/1  "<TaillightRight>"
  Bus Selector/32 -> Pwr23/1  "<CabLight1>"
  Bus Selector/33 -> Pwr32/1  "<CabLight2>"
  Bus Selector/34 -> Pwr33/1  "<BrakeCylinderPressure>"
  Bus Selector/35 -> Pwr34/1  "<MainReservoirPipePressure>"
  Bus Selector1/35 -> Pwr63/1  "<MainReservoirPipePressure>"
  Bus Selector1/34 -> Pwr62/1  "<BrakeCylinderPressure>"
  Bus Selector1/33 -> Pwr61/1  "<CabLight2>"
  Bus Selector1/32 -> Pwr51/1  "<CabLight1>"
  Bus Selector1/31 -> Pwr50/1  "<TaillightRight>"
  Bus Selector1/30 -> Pwr49/1  "<TaillightLeft>"
  Bus Selector1/29 -> Pwr48/1  "<HeadlightRight>"
  Bus Selector1/28 -> Pwr46/1  "<HeadlightLeft>"
  Bus Selector1/27 -> Pwr45/1  "<DoorNotClosedLight2>"
  Bus Selector1/26 -> Pwr60/1  "<DoorNotClosedLight1>"
  Bus Selector1/25 -> Pwr59/1  "<PneumaticBrakesNotReleasedLight2>"
  Bus Selector1/24 -> Pwr57/1  "<PneumaticBrakesNotReleasedLight1>"
  Bus Selector1/23 -> Pwr56/1  "<OverheadLineVoltageGaugeBacklight>"
  Bus Selector1/22 -> Pwr55/1  "<OverheadLineVoltageGauge>"
  Bus Selector1/21 -> Pwr54/1  "<DualBatteryVoltageGaugeBacklight>"
  Bus Selector1/20 -> Pwr53/1  "<Battery220VVoltageGauge>"
  Bus Selector1/19 -> Pwr52/1  "<Battery110VVoltageGauge>"
  Bus Selector1/18 -> Pwr44/1  "<ParkBrakeApplyPBLight>"
  Bus Selector1/17 -> Pwr43/1  "<PantoDownPBLight>"
  Bus Selector1/16 -> Pwr42/1  "<PantoUpPBLight>"
  Bus Selector1/15 -> Pwr41/1  "<TCMSAlarmBuzzer>"
  Bus Selector1/14 -> Pwr40/1  "<VigilanceBuzzer>"
  Bus Selector1/13 -> Pwr39/1  "<DualPressureGaugeBacklight>"
  Bus Selector1/12 -> Pwr38/1  "<BrakeCylinderPressureGauge>"
  Bus Selector1/11 -> Pwr37/1  "<MainReservoirPipePressureGauge>"
  Bus Selector1/10 -> Pwr69/1  "<ATOStartPBLight>"
  Bus Selector1/9 -> Pwr68/1  "<EmergencyBrakePBLight>"
  Bus Selector1/8 -> Pwr67/1  "<EmergencyBrakeAppliedLight>"
  Bus Selector1/7 -> Pwr66/1  "<AllDoorsClosedLight>"
  Bus Selector1/6 -> Pwr65/1  "<HSCBClosePBLight>"
  Bus Selector1/5 -> Pwr64/1  "<LeftDoorOpenPBLight2>"
  Bus Selector1/4 -> Pwr58/1  "<LeftDoorOpenPBLight1>"
  Bus Selector1/3 -> Pwr47/1  "<RightDoorOpenPBLight2>"
  Bus Selector1/2 -> Pwr36/1  "<RightDoorOpenPBLight1>"
  Bus Selector1/1 -> Pwr35/1  "<AutomaticChangeEndPBLight>"
  Selector2/1 -> Bus Selector1/1
  SetValue2/1 -> Selector2/2

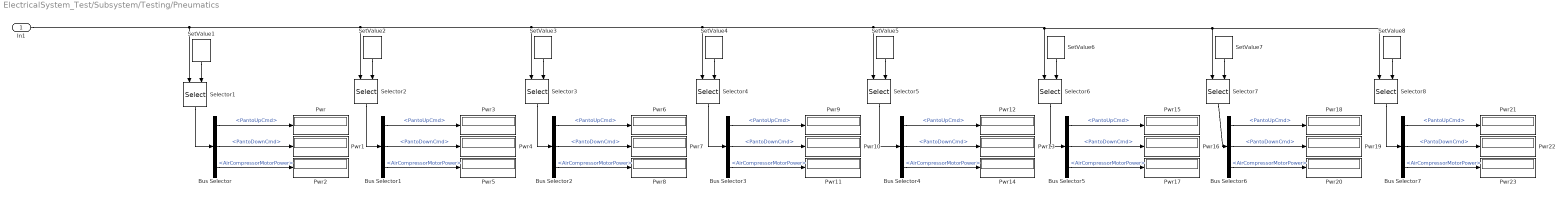
== system ElectricalSystem_Test/Subsystem/Testing/Pneumatics ==
  In1 : Inport
  Bus Selector{,1..7} (8 alike) : BusSelector  OutputSignals=Pneumatics.PantoUpCmd,Pneumatics.PantoDownCmd,Pneumatics.AirCompressorMotorPower
  Pwr{,1..23} (24 alike) : Display
  Selector{1..8} (8 alike) : Selector  InputPortWidth=8  IndexOptions=Index vector (port)  Indices=[1 3]  OutputSizes=1
  SetValue1 : TestBenchLib/SetValue  value=1  init_value=1  WorkspaceVarName=0
      settings: SourceProductName=Sydac Utilities
  SetValue2 : TestBenchLib/SetValue  value=2  init_value=2  WorkspaceVarName=0
      settings: SourceProductName=Sydac Utilities
  SetValue3 : TestBenchLib/SetValue  value=3  init_value=3  WorkspaceVarName=0
      settings: SourceProductName=Sydac Utilities
  SetValue4 : TestBenchLib/SetValue  value=4  init_value=4  WorkspaceVarName=0
      settings: SourceProductName=Sydac Utilities
  SetValue5 : TestBenchLib/SetValue  value=5  init_value=5  WorkspaceVarName=0
      settings: SourceProductName=Sydac Utilities
  SetValue6 : TestBenchLib/SetValue  value=6  init_value=6  WorkspaceVarName=0
      settings: SourceProductName=Sydac Utilities
  SetValue7 : TestBenchLib/SetValue  value=7  init_value=7  WorkspaceVarName=0
      settings: SourceProductName=Sydac Utilities
  SetValue8 : TestBenchLib/SetValue  value=8  init_value=8  WorkspaceVarName=0
      settings: SourceProductName=Sydac Utilities
  wires:
  Selector5/1 -> Bus Selector4/1
  Selector7/1 -> Bus Selector6/1
  Selector6/1 -> Bus Selector5/1
  Selector3/1 -> Bus Selector2/1
  SetValue8/1 -> Selector8/2
  SetValue7/1 -> Selector7/2
  SetValue6/1 -> Selector6/2
  In1/1 -> Selector1/1, Selector2/1, Selector3/1, Selector4/1, Selector5/1, Selector6/1, Selector7/1, Selector8/1
  SetValue5/1 -> Selector5/2
  SetValue4/1 -> Selector4/2
  SetValue3/1 -> Selector3/2
  SetValue2/1 -> Selector2/2
  Selector2/1 -> Bus Selector1/1
  Bus Selector/3 -> Pwr2/1  "<AirCompressorMotorPower>"
  Bus Selector/2 -> Pwr1/1  "<PantoDownCmd>"
  Bus Selector/1 -> Pwr/1  "<PantoUpCmd>"
  SetValue1/1 -> Selector1/2
  Selector1/1 -> Bus Selector/1
  Bus Selector1/2 -> Pwr4/1  "<PantoDownCmd>"
  Bus Selector1/1 -> Pwr3/1  "<PantoUpCmd>"
  Bus Selector1/3 -> Pwr5/1  "<AirCompressorMotorPower>"
  Bus Selector2/2 -> Pwr7/1  "<PantoDownCmd>"
  Bus Selector2/1 -> Pwr6/1  "<PantoUpCmd>"
  Bus Selector2/3 -> Pwr8/1  "<AirCompressorMotorPower>"
  Bus Selector3/2 -> Pwr10/1  "<PantoDownCmd>"
  Bus Selector3/1 -> Pwr9/1  "<PantoUpCmd>"
  Bus Selector3/3 -> Pwr11/1  "<AirCompressorMotorPower>"
  Selector4/1 -> Bus Selector3/1
  Bus Selector4/2 -> Pwr13/1  "<PantoDownCmd>"
  Bus Selector4/1 -> Pwr12/1  "<PantoUpCmd>"
  Bus Selector4/3 -> Pwr14/1  "<AirCompressorMotorPower>"
  Bus Selector5/2 -> Pwr16/1  "<PantoDownCmd>"
  Bus Selector5/1 -> Pwr15/1  "<PantoUpCmd>"
  Bus Selector5/3 -> Pwr17/1  "<AirCompressorMotorPower>"
  Bus Selector6/2 -> Pwr19/1  "<PantoDownCmd>"
  Bus Selector6/1 -> Pwr18/1  "<PantoUpCmd>"
  Bus Selector6/3 -> Pwr20/1  "<AirCompressorMotorPower>"
  Bus Selector7/2 -> Pwr22/1  "<PantoDownCmd>"
  Bus Selector7/1 -> Pwr21/1  "<PantoUpCmd>"
  Bus Selector7/3 -> Pwr23/1  "<AirCompressorMotorPower>"
  Selector8/1 -> Bus Selector7/1
